simulink model "VCMGCM1962020b_v2"  (R2020b)
settings: Solver=FixedStepDiscrete  StartTime=0.0  StopTime=10.0  FixedStep=0.005  RelTol=1e-3  EnableMultiTasking=on
PreLoadFcn:
  | try, model_open; catch, disp('Error occurred while executing model pre-load callback: model_open.m'); disp('Please assure that the MATLAB working directory is set to the model directory before opening.'); end
InitFcn:
  | try, model_open; catch, end
undefined symbols (not defined in the file): Bridge, GCM, H, raptor_get_param_eval, raptor_get_safe_string, raptor_xcp_function
libraries: Blocks_lib x1165, Raptor_lib x665, simulink x62, VCM_lib x5
(part 2 of 23)

== system VCMGCM1962020b_v2/Fgnd/Diagnostics/Fault Statuses ==
  Data : Inport
  Clear All Faults : Subsystem
  Drive Cycle Logic : Subsystem
  FCC(w/Inpt) : Blocks_lib/FCC(w//Inpt)  SystemSampleTime=-1  VariantActivationTime=update diagram  Latency=0  AutoFrameSizeCalculation=off
  FltStatuses : Blocks_lib/FltStatuses  nam='Fault1'  group=[group ' | Fault1']
  FltStatuses1 : Blocks_lib/FltStatuses  nam='Fault2'  group=[group ' | Fault2']
  FltStatuses2 : Blocks_lib/FltStatuses  nam='Fault3'  group=[group ' | Fault3']
  Header : Blocks_lib/Header  width=Portrait  addtext=''
  Save NV : Subsystem
  Status Marquees : Subsystem
  raptor_adjustment : Raptor_lib/Data Storage/raptor_adjustment  paramName='FaultMarqueeRate'  nameSource=Parameter  initValue=1/samptime  dataType=uint16  storage=Calibration  calDispType=Number  calEnum={'Disabled', 'Enabled'}  calGain=samptime  calOffset=0  calMax=inf  calMin=-inf  calFormat='0.3'  calUnit='sec'  calHelp='Fault marquee update rate'  calAccess=1  calFunction=group  calDispHeaders=off  calColHeaders={'Col1' 'Col2' 'Col3'}  calRowHeaders={'Row1' 'Row2' 'Row3'}
      settings: SourceProductName=Raptor
  raptor_data_def1 : Raptor_lib/Data Storage/raptor_data_def  dataName='ClearFaults'  initValue=0  dataType=boolean  storage=Volatile (RAM)  calVisible=on  calType=Adjustment  calDispType=Enumeration  calEnum={'-', 'Clear'}  calGain=1  calOffset=0  calMin=-inf  calMax=inf  calFormat=''  calUnit='enum'  calHelp='Clear faults'  calAccess=1  calFunction=group  calDispHeaders=off  calColHeaders={'Col1' 'Col2' 'Col3'}  calRowHeaders={'Row1' 'Row2' 'Row3'}
      settings: SourceProductName=Raptor
  raptor_data_def2 : Raptor_lib/Data Storage/raptor_data_def  dataName='SaveNV'  initValue=0  dataType=boolean  storage=Volatile (RAM)  calVisible=on  calType=Adjustment  calDispType=Enumeration  calEnum={'-', 'Save'}  calGain=1  calOffset=0  calMin=-inf  calMax=inf  calFormat=''  calUnit='enum'  calHelp='Save nonvolatile'  calAccess=1  calFunction=group  calDispHeaders=off  calColHeaders={'Col1' 'Col2' 'Col3'}  calRowHeaders={'Row1' 'Row2' 'Row3'}
      settings: SourceProductName=Raptor
  raptor_data_read : Raptor_lib/Data Storage/raptor_data_read  dataName='ClearFaults'  dataShape=Scalar  idxSource=Input  idxRow=1  idxCol=1
      settings: SourceProductName=Raptor
  raptor_data_read1 : Raptor_lib/Data Storage/raptor_data_read  dataName='SaveNV'  dataShape=Scalar  idxSource=Input  idxRow=1  idxCol=1
      settings: SourceProductName=Raptor
  raptor_measurement : Raptor_lib/Data Storage/raptor_measurement  paramName='NVStoreInProgress'  nameSource=Parameter  calDispType=Number  calEnum={'Disabled', 'Enabled'}  calGain=1  calOffset=0  calMax=inf  calMin=-inf  calFormat=''  calUnit='Bool'  calHelp='Nonvolatile store in progress'  calAccess=1  calFunction='Diagnostics | Fault Statuses'  calVisible=on
      settings: SourceProductName=Raptor
  raptor_measurement1 : Raptor_lib/Data Storage/raptor_measurement  paramName='NVSucceeded'  nameSource=Parameter  calDispType=Number  calEnum={'Disabled', 'Enabled'}  calGain=1  calOffset=0  calMax=inf  calMin=-inf  calFormat=''  calUnit='Bool'  calHelp='Nonvolatile store succeeded'  calAccess=1  calFunction='Diagnostics | Fault Statuses'  calVisible=on
      settings: SourceProductName=Raptor
  raptor_sfun_nv_status : Raptor_lib/Data Storage/raptor_sfun_nv_status  showStatus=Store In Progess
      settings: SourceProductName=Raptor
  raptor_sfun_nv_status1 : Raptor_lib/Data Storage/raptor_sfun_nv_status  showStatus=Store Succeeded
      settings: SourceProductName=Raptor
  wires:
  raptor_adjustment/1 -> FCC(w/Inpt)/1
  raptor_data_read/1 -> Clear All Faults/Enable
  raptor_data_read1/1 -> Save NV/Enable
  FCC(w/Inpt)/1 -> Status Marquees/Trigger
  Data/1 -> Drive Cycle Logic/1(Data)
  raptor_sfun_nv_status/1 -> raptor_measurement/1
  raptor_sfun_nv_status1/1 -> raptor_measurement1/1

== system VCMGCM1962020b_v2/Fgnd/Sensors/CAN ==
  Data : Inport
  Battery : Subsystem  mask{bus='CAN1'}
      mask prompts: bus "CAN Bus"
      mask Display: disp(['BMS: Battery\n' bus]);
  Bus Creator : BusCreator  Inputs=5
  CCS Interface : Subsystem  Commented=on  mask{nam='CCS', bus='CAN1'}
      mask prompts: nam "Name"; bus "CAN Bus"
      mask Display: disp(['CCS Interface: IoTecha M2iEV\n' nam '\n' bus]);
  Charger : Subsystem  mask{nam='Chgr', bus='CAN1'}
      mask prompts: nam "Name"; bus "CAN Bus"
      mask Display: disp(['On-Board Charger: Dilong\n' nam '\n' bus]);
  DC/DC Converter : Subsystem  mask{nam='DCDC', bus='CAN1'}
      mask prompts: nam "Name"; bus "CAN Bus"
      mask Display: disp(['DC/DC Converter: Dilong\n' nam '\n' bus]);
  Header : Blocks_lib/Header  width=Portrait  addtext=''
  Inverter : Subsystem  mask{bus='CAN3'}
      mask prompts: bus "CAN Bus"
      mask Display: disp(['Sieatta: Invrtr2\n' bus]);
  Other : Subsystem
  CAN : Outport  VectorParamsAs1DForOutWhenUnconnected=off
  wires:
  Inverter/1(CAN) -> Bus Creator/4
  Other/1(CAN) -> Bus Creator/5
  Charger/1(CAN) -> Bus Creator/2
  Battery/1(CAN) -> Bus Creator/1
  Bus Creator/1 -> CAN/1  "CAN"
  Data/1 -> Battery/1(Data), CCS Interface/1(Data), Charger/1(Data), Other/1(Data), Inverter/1(Data), DC/DC Converter/1(Data)
  DC/DC Converter/1(CAN) -> Bus Creator/3

== system VCMGCM1962020b_v2/Fgnd/Sensors/Sensors ==
  Data : Inport
  Bus Creator : BusCreator  Inputs=3
  Driver Inputs : Subsystem
  Header : Blocks_lib/Header  width=Portrait  addtext=''
  Other : Subsystem
  Voltage : Subsystem
  Sns : Outport  VectorParamsAs1DForOutWhenUnconnected=off
  wires:
  Other/1(Sns) -> Bus Creator/3
  Driver Inputs/1(Sns) -> Bus Creator/2
  Voltage/1(Sns) -> Bus Creator/1
  Bus Creator/1 -> Sns/1  "Sensors"
  Data/1 -> Voltage/1(Data), Other/1(Data), Driver Inputs/1(Data)

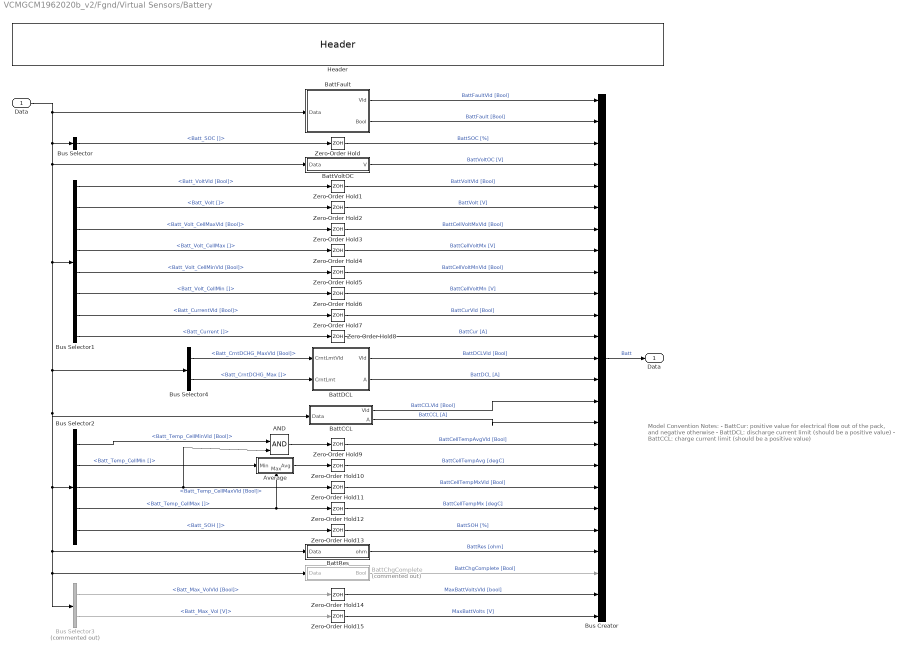
== system VCMGCM1962020b_v2/Fgnd/Virtual Sensors/Battery ==
  note: Model Convention Notes:
      | - BattCur: positive value for electrical flow out of the pack, and negative otherwise
      | - BattDCL: discharge current limit (should be a positive value)
      | - BattCCL: charge current limit (should be a positive value)
  Data : Inport
  AND : Logic  IconShape=distinctive  AllPortsSameDT=off  OutDataTypeStr=boolean
  Average : Subsystem
      settings: PortSchema="{\"entries\":[{\"content\":{\"sides\":[{\"content\":{\"connectorIds\":[\"In1\"]},\"type\":\"ConnectorPlacement.EquallySpacedRectSide\",\"uuid\":\"d9ce9f9a-84a0-4d2c-b22c-bde2c1e2d059\"},{\"content\":{\"connectorIds\":[\"Out1\"],\"side\":\"RIGHT\"},\"type\":\"ConnectorPlacement.EquallySpacedRectSide\",\"uuid\":\"15af732b-6599-4303-92ae-4f716d2d6ef7\"},{\"content\":{\"connectorIds\":[],\"side\":\"TOP\"},\"type\":\"ConnectorPlacement.EquallySpacedRectSide\",\"uuid\":\"c502e606-7455-4b79-ae1a-42fe114835b7\"},{\"content\":{\"connectorIds\":[\"In2\"],\"side\":\"BOTTOM\"},\"type\":\"ConnectorPlacement.EquallySpacedRectSide\",\"uuid\":\"09754e92-d425-4c42-b1f4-651282dd1591\"},{\"content\":{\"connectorIds\":[],\"side\":\"HIDDEN\"},\"type\":\"ConnectorPlacement.EquallySpacedRectSide\",\"uuid\":\"b5cad8d8-bd34-4b5c-af02-955cb15cf870\"}]},\"type\":\"ConnectorPlacement.EquallySpacedConnector\",\"uuid\":\"2eb02162-2dec-4f79-8472-1f908402e422\"}],\"packageUris\":[\"http://schema.mathworks.com/mf0/Connector/R2020b\"],\"version\":\"1.0\"}"
  BattCCL : Subsystem
  BattChgComplete : Subsystem  Commented=on
  BattDCL : Subsystem
  BattFault : Subsystem
  BattRes : Subsystem
  BattVoltOC : Subsystem
  Bus Creator : BusCreator  Inputs=25
  Bus Selector : BusSelector  OutputSignals=Sensors.CAN.Batt.BMS2_VoltageSOC.Batt_SOC.Batt_SOC []
  Bus Selector1 : BusSelector  OutputSignals=Sensors.CAN.Batt.BMS2_VoltageSOC.Batt_Volt.Batt_VoltVld [Bool],Sensors.CAN.Batt.BMS2_VoltageSOC.Batt_Volt.Batt_Volt [],Sensors.CAN.Batt.BMS3_Cell.Batt_Volt_CellMax.Batt_Volt_CellMaxVld [Bool],Sensors.CAN.Batt.BMS3_Cell.Batt_Volt_CellMax.Batt_Volt_CellMax [],Sensors.CAN.Batt.BMS3_Cell.Batt_Volt_CellMin.Batt_Volt_CellMinVld [Bool],Sensors.CAN.Batt.BMS3_Cell.Batt_Volt_CellMin.Batt_Volt_CellMin [],Sensors.CAN.Batt.BMS1_Currents.Batt_Current.Batt_CurrentVld [Bool],Sensors.CAN.Batt.BMS1_Currents.Batt_Current.Batt_Current []
  Bus Selector2 : BusSelector  OutputSignals=Sensors.CAN.Batt.BMS3_Cell.Batt_Temp_CellMin.Batt_Temp_CellMinVld [Bool],Sensors.CAN.Batt.BMS3_Cell.Batt_Temp_CellMin.Batt_Temp_CellMin [],Sensors.CAN.Batt.BMS3_Cell.Batt_Temp_CellMax.Batt_Temp_CellMaxVld [Bool],Sensors.CAN.Batt.BMS3_Cell.Batt_Temp_CellMax.Batt_Temp_CellMax [],Sensors.CAN.Batt.BMS2_VoltageSOC.Batt_SOH.Batt_SOH []
  Bus Selector3 : BusSelector  Commented=on  OutputSignals=Sensors.CAN.Batt.HVES1_Data7.Batt_Max_Vol.Batt_Max_VolVld [Bool],Sensors.CAN.Batt.HVES1_Data7.Batt_Max_Vol.Batt_Max_Vol [V]
  Bus Selector4 : BusSelector  OutputSignals=Sensors.CAN.Batt.BMS1_Currents.Batt_CrntDCHG_Max.Batt_CrntDCHG_MaxVld [Bool],Sensors.CAN.Batt.BMS1_Currents.Batt_CrntDCHG_Max.Batt_CrntDCHG_Max []
  Header : Blocks_lib/Header  width=Portrait  addtext=''
  Zero-Order Hold{,1..15} (16 alike) : ZeroOrderHold  SampleTime=-1
  " Data" : Outport  VectorParamsAs1DForOutWhenUnconnected=off
  wires:
  Zero-Order Hold13/1 -> Bus Creator/21  "BattSOH [%]"
  BattRes/1(ohm) -> Bus Creator/22  "BattRes [ohm]"
  BattChgComplete/1(Bool) -> Bus Creator/23  "BattChgComplete [Bool]"
  Zero-Order Hold12/1 -> Bus Creator/20  "BattCellTempMx [degC]"
  Zero-Order Hold10/1 -> Bus Creator/18  "BattCellTempAvg [degC]"
  BattCCL/2(A) -> Bus Creator/16  "BattCCL [A]"
  BattDCL/2(A) -> Bus Creator/14  "BattDCL [A]"
  Zero-Order Hold8/1 -> Bus Creator/12  "BattCur [A]"
  Zero-Order Hold6/1 -> Bus Creator/10  "BattCellVoltMn [V]"
  Zero-Order Hold4/1 -> Bus Creator/8  "BattCellVoltMx [V]"
  Zero-Order Hold2/1 -> Bus Creator/6  "BattVolt [V]"
  Bus Creator/1 -> " Data"/1  "Batt"
  Zero-Order Hold/1 -> Bus Creator/3  "BattSOC [%]"
  Bus Selector/1 -> Zero-Order Hold/1  "<Batt_SOC []>"
  BattVoltOC/1(V) -> Bus Creator/4  "BattVoltOC [V]"
  Data/1 -> BattVoltOC/1(Data), BattRes/1(Data), Bus Selector3/1, BattChgComplete/1(Data), Bus Selector2/1, BattCCL/1(Data), Bus Selector4/1, Bus Selector1/1, Bus Selector/1, BattFault/1(Data)
  BattFault/1(Vld) -> Bus Creator/1  "BattFaultVld [Bool]"
  Zero-Order Hold1/1 -> Bus Creator/5  "BattVoltVld [Bool]"
  Bus Selector1/7 -> Zero-Order Hold7/1  "<Batt_CurrentVld [Bool]>"
  Bus Selector1/6 -> Zero-Order Hold6/1  "<Batt_Volt_CellMin []>"
  Bus Selector1/5 -> Zero-Order Hold5/1  "<Batt_Volt_CellMinVld [Bool]>"
  Bus Selector1/4 -> Zero-Order Hold4/1  "<Batt_Volt_CellMax []>"
  Bus Selector1/3 -> Zero-Order Hold3/1  "<Batt_Volt_CellMaxVld [Bool]>"
  Bus Selector1/2 -> Zero-Order Hold2/1  "<Batt_Volt []>"
  Bus Selector1/1 -> Zero-Order Hold1/1  "<Batt_VoltVld [Bool]>"
  Zero-Order Hold3/1 -> Bus Creator/7  "BattCellVoltMxVld [Bool]"
  Zero-Order Hold5/1 -> Bus Creator/9  "BattCellVoltMnVld [Bool]"
  Zero-Order Hold7/1 -> Bus Creator/11  "BattCurVld [Bool]"
  BattDCL/1(Vld) -> Bus Creator/13  "BattDCLVld [Bool]"
  BattCCL/1(Vld) -> Bus Creator/15  "BattCCLVld [Bool]"
  Zero-Order Hold9/1 -> Bus Creator/17  "BattCellTempAvgVld [Bool]"
  Zero-Order Hold11/1 -> Bus Creator/19  "BattCellTempMxVld [Bool]"
  BattFault/2(Bool) -> Bus Creator/2  "BattFault [Bool]"
  Bus Selector3/1 -> Zero-Order Hold14/1  "<Batt_Max_VolVld [Bool]>"
  Bus Selector3/2 -> Zero-Order Hold15/1  "<Batt_Max_Vol [V]>"
  Zero-Order Hold15/1 -> Bus Creator/25  "MaxBattVolts [V]"
  Zero-Order Hold14/1 -> Bus Creator/24  "MaxBattVoltsVld [bool]"
  AND/1 -> Zero-Order Hold9/1
  Bus Selector2/1 -> AND/1  "<Batt_Temp_CellMinVld [Bool]>"
  Bus Selector2/2 -> Average/1(Min)  "<Batt_Temp_CellMin []>"
  Bus Selector2/3 -> AND/2, Zero-Order Hold11/1  "<Batt_Temp_CellMaxVld [Bool]>"
  Bus Selector2/4 -> Zero-Order Hold12/1, Average/2(Max)  "<Batt_Temp_CellMax []>"
  Bus Selector2/5 -> Zero-Order Hold13/1  "<Batt_SOH []>"
  Average/1(Avg) -> Zero-Order Hold10/1
  Bus Selector4/1 -> BattDCL/1(CrntLmtVld)  "<Batt_CrntDCHG_MaxVld [Bool]>"
  Bus Selector4/2 -> BattDCL/2(CrntLmt)  "<Batt_CrntDCHG_Max []>"
  Bus Selector1/8 -> Zero-Order Hold8/1  "<Batt_Current []>"

== system VCMGCM1962020b_v2/Fgnd/Virtual Sensors/Charger ==
  Data : Inport
  Bus Creator : BusCreator  Inputs=4
  ChgPlugState : Subsystem
  ChgPortDCVolt : Subsystem
  Header : Blocks_lib/Header  width=Portrait  addtext=''
  Off Board : Subsystem  Commented=on
  On Board : Subsystem
  " Data" : Outport  VectorParamsAs1DForOutWhenUnconnected=off
  wires:
  Bus Creator/1 -> " Data"/1  "Chgr"
  ChgPlugState/1(enum) -> Bus Creator/1  "ChgPlugState [enum]"
  On Board/1(" Data") -> Bus Creator/4  "OnBoard"
  ChgPortDCVolt/1(Vld) -> Bus Creator/2  "ChgPortDCVoltVld [Bool]"
  ChgPortDCVolt/2(V) -> Bus Creator/3  "ChgPortDCVolt [V]"
  Data/1 -> ChgPlugState/1(Data), On Board/1(Data), Off Board/1(Data), ChgPortDCVolt/1(Data)

== system VCMGCM1962020b_v2/Fgnd/Virtual Sensors/DC//DC Converter ==
  Data : Inport
  Bus Creator : BusCreator  Inputs=6
  Bus Selector : BusSelector  OutputSignals=Sensors.CAN.DCDC.DCDC_Status_0_16V.DCDCOutput_Voltage_0_16V.DCDCOutput_Voltage_0_16VVld [Bool],Sensors.CAN.DCDC.DCDC_Status_0_16V.DCDCOutput_Voltage_0_16V.DCDCOutput_Voltage_0_16V [V]
  Bus Selector1 : BusSelector  OutputSignals=Sensors.CAN.DCDC.DCDC_Status_0_16V.DCDC_Inner_temp_0_16V.DCDC_Inner_temp_0_16V [C]
  DCDCFault : Subsystem
  DCDCInptCur : Subsystem
  Header : Blocks_lib/Header  width=Portrait  addtext=''
  Zero-Order Hold : ZeroOrderHold  SampleTime=-1
  Zero-Order Hold1 : ZeroOrderHold  SampleTime=-1
  Zero-Order Hold2 : ZeroOrderHold  SampleTime=-1
  " Data" : Outport  VectorParamsAs1DForOutWhenUnconnected=off
  wires:
  Bus Creator/1 -> " Data"/1  "DCDC"
  Zero-Order Hold2/1 -> Bus Creator/6  "DCDCTemp [degC]"
  Zero-Order Hold1/1 -> Bus Creator/4  "DCDCInptVolt [V]"
  Bus Selector1/1 -> Zero-Order Hold2/1  "<DCDC_Inner_temp_0_16V [C]>"
  Bus Selector/2 -> Zero-Order Hold1/1  "<DCDCOutput_Voltage_0_16V [V]>"
  Zero-Order Hold/1 -> Bus Creator/3  "DCDCInptVoltVld [Bool]"
  Bus Selector/1 -> Zero-Order Hold/1  "<DCDCOutput_Voltage_0_16VVld [Bool]>"
  DCDCFault/1(Vld) -> Bus Creator/1  "DCDCFaultVld [Bool]"
  Data/1 -> DCDCFault/1(Data), Bus Selector/1, Bus Selector1/1, DCDCInptCur/1(Data)
  DCDCFault/2(Bool) -> Bus Creator/2  "DCDCFault [Bool]"
  DCDCInptCur/1(A) -> Bus Creator/5  "DCDCInptCur [A]"

== system VCMGCM1962020b_v2/Fgnd/Virtual Sensors/Drive Inverter ==
  note: TBC
  note: Model Convention Notes:
      | - InvtrCur: positive value for electrical flow into the inverter, and negative otherwise
      | - MtrTrq: may be positive or negative (motoring when torque and speed have same signs; generating when torque and speed have opposite signs)
      | - MtrTrqLimMx: limit on torque in positive speed direction (should be a positive value)
      | - MtrTrqLimMn: limit on torque in negative speed direction (should be a negative value)
  Data : Inport
  Bus Creator : BusCreator  Inputs=16
  Bus Selector : BusSelector  OutputSignals=Sensors.CAN.DrvInvtr.EM3.EM3DCv.EM3_InverterDcV.EM3_InverterDcVVld [Bool],Sensors.CAN.DrvInvtr.EM3.EM3DCv.EM3_InverterDcV.EM3_InverterDcV [V]
  Bus Selector1 : BusSelector  OutputSignals=Sensors.CAN.DrvInvtr.EM2.EM2Invemp.EM2_InverterBridgeMaxTemp.EM2_InverterBridgeMaxTemp [degC],Sensors.CAN.DrvInvtr.EM4.EM4Spd.EM4_SpdAct.EM4_SpdActVld [Bool],Sensors.CAN.DrvInvtr.EM4.EM4Spd.EM4_SpdAct.EM4_SpdAct [rpm],Sensors.CAN.DrvInvtr.EM4.EM4Trq.EM4_TorqAct.EM4_TorqActVld [Bool],Sensors.CAN.DrvInvtr.EM4.EM4Trq.EM4_TorqAct.EM4_TorqAct [Nm],Sensors.CAN.DrvInvtr.EM1.EM1_eBridgeOvrTemp.EM1_eBridgeOvrTempVld [Bool],Sensors.CAN.DrvInvtr.EM1.EM1_eMotorOvrTemp.EM1_eMotorOvrTemp []
  Constant : Constant  Value=double(99999)
  DrvInvtrCur : Subsystem
  DrvInvtrFault : Subsystem
  DrvMtrTmp : Subsystem
  Gain : Gain  Gain=-1
  Header : Blocks_lib/Header  width=Portrait  addtext=''
  Zero-Order Hold{,1..10} (11 alike) : ZeroOrderHold  SampleTime=-1
  " Data" : Outport  VectorParamsAs1DForOutWhenUnconnected=off
  wires:
  Bus Creator/1 -> " Data"/1  "DrvInvtr"
  Zero-Order Hold1/1 -> Bus Creator/4  "DrvInvtrVolt [V]"
  Zero-Order Hold2/1 -> Bus Creator/7  "DrvInvtrTemp [degC]"
  DrvMtrTmp/1(degC) -> Bus Creator/16  "DrvMtrTemp [degC]"
  Zero-Order Hold8/1 -> Bus Creator/13  "DrvMtrTrqLimMn [Nm]"
  Zero-Order Hold4/1 -> Bus Creator/9  "DrvMtrSpd [rpm]"
  Zero-Order Hold7/1 -> Bus Creator/12  "DrvMtrTrqLimMx [Nm]"
  Bus Selector/2 -> Zero-Order Hold1/1  "<EM3_InverterDcV [V]>"
  Constant/1 -> Gain/1, Zero-Order Hold7/1  "<DrvInvtrNegativeTorqueAvailable [Nm]>"
  Zero-Order Hold6/1 -> Bus Creator/11  "DrvMtrTrq [Nm]"
  Zero-Order Hold5/1 -> Bus Creator/10  "DrvMtrTrqVld [Bool]"
  Bus Selector/1 -> Zero-Order Hold/1  "<EM3_InverterDcVVld [Bool]>"
  Zero-Order Hold/1 -> Bus Creator/3  "DrvInvtrVoltVld [Bool]"
  DrvInvtrCur/1(Vld) -> Bus Creator/5  "DrvInvtrCurVld [Bool]"
  DrvInvtrFault/1(Vld) -> Bus Creator/1  "DrvInvtrFaultVld [Bool]"
  Data/1 -> DrvInvtrFault/1(Data), Bus Selector/1, DrvMtrTmp/1(Data), Bus Selector1/1, DrvInvtrCur/1(Data)
  Zero-Order Hold3/1 -> Bus Creator/8  "DrvMtrSpdVld [Bool]"
  DrvInvtrFault/2(Bool) -> Bus Creator/2  "DrvInvtrFault [Bool]"
  DrvInvtrCur/2(A) -> Bus Creator/6  "DrvInvtrCur [A]"
  Gain/1 -> Zero-Order Hold8/1
  Zero-Order Hold9/1 -> Bus Creator/14  "DrvInvtrOvrTemp [Bool]"
  Zero-Order Hold10/1 -> Bus Creator/15  "DrvMtrOvrTemp [Bool]"
  Bus Selector1/1 -> Zero-Order Hold2/1  "<EM2_InverterBridgeMaxTemp [degC]>"
  Bus Selector1/2 -> Zero-Order Hold3/1  "<EM4_SpdActVld [Bool]>"
  Bus Selector1/3 -> Zero-Order Hold4/1  "<EM4_SpdAct [rpm]>"
  Bus Selector1/4 -> Zero-Order Hold5/1  "<EM4_TorqActVld [Bool]>"
  Bus Selector1/5 -> Zero-Order Hold6/1  "<EM4_TorqAct [Nm]>"
  Bus Selector1/6 -> Zero-Order Hold9/1  "<EM1_eBridgeOvrTempVld [Bool]>"
  Bus Selector1/7 -> Zero-Order Hold10/1  "<EM1_eMotorOvrTemp []>"

== system VCMGCM1962020b_v2/Fgnd/Virtual Sensors/Driver Inputs ==
  Data : Inport
  APP : Subsystem
  Brk : Subsystem
  Bus Creator : BusCreator  Inputs=15
  Bus Selector : BusSelector  OutputSignals=Sensors.Sensors.Driver.Rev.Rev [Bool],Sensors.Sensors.Driver.Ntrl.Ntrl [Bool],Sensors.Sensors.Driver.Drv.Drv [Bool],Sensors.Sensors.Driver.CCOn.CCOn [Bool],Sensors.Sensors.Driver.CCCancel.CCCancel [Bool],Sensors.Sensors.Driver.CCSetCst.CCSetCst [Bool],Sensors.Sensors.Driver.CCRsmAcc.CCRsmAcc [Bool]
  Header : Blocks_lib/Header  width=Portrait  addtext=''
  NOR : Logic  Operator=NOR  AllPortsSameDT=off  OutDataTypeStr=boolean
  ParkBrake : Subsystem
  Terminator : Terminator
  VehPwrMode : Subsystem
  Zero-Order Hold{1..8} (8 alike) : ZeroOrderHold  SampleTime=-1
  " Data" : Outport  VectorParamsAs1DForOutWhenUnconnected=off
  wires:
  APP/1(Vld) -> Bus Creator/2  "APPVld [Bool]"
  Bus Selector/6 -> Zero-Order Hold7/1  "<CCSetCst [Bool]>"
  Bus Selector/5 -> Zero-Order Hold6/1  "<CCCancel [Bool]>"
  Bus Selector/4 -> Zero-Order Hold5/1  "<CCOn [Bool]>"
  Bus Selector/3 -> NOR/2, Zero-Order Hold4/1  "<Drv [Bool]>"
  Bus Selector/1 -> Zero-Order Hold2/1, NOR/1  "<Rev [Bool]>"
  Data/1 -> VehPwrMode/1(Data), ParkBrake/1(Data), Bus Selector/1, Brk/1(Data), APP/1(Data)
  Bus Creator/1 -> " Data"/1  "Driver"
  Zero-Order Hold6/1 -> Bus Creator/13  "CCCancel [Bool]"
  Zero-Order Hold5/1 -> Bus Creator/12  "CCOn [Bool]"
  Zero-Order Hold8/1 -> Bus Creator/15  "CCRsmAcc [Bool]"
  Zero-Order Hold7/1 -> Bus Creator/14  "CCSetCst [Bool]"
  Zero-Order Hold4/1 -> Bus Creator/11  "Drv [Bool]"
  Zero-Order Hold3/1 -> Bus Creator/10  "Ntrl [Bool]"
  Zero-Order Hold2/1 -> Bus Creator/9  "Rev [Bool]"
  Zero-Order Hold1/1 -> Bus Creator/8  "Prk [Bool]"
  VehPwrMode/1(enum) -> Bus Creator/1  "VehPwrMode [enum]"
  APP/2(%) -> Bus Creator/3  "APP [%]"
  Brk/2(Brk) -> Bus Creator/5  "BrkSw [Bool]"
  Bus Selector/7 -> Zero-Order Hold8/1  "<CCRsmAcc [Bool]>"
  Brk/1(Vld) -> Bus Creator/4  "BrkVld [Bool]"
  Brk/3(Pos) -> Bus Creator/6  "BrkPos [%]"
  Brk/4(PosVld) -> Bus Creator/7  "BrkPosVld [Bool]"
  NOR/1 -> Zero-Order Hold3/1
  Bus Selector/2 -> Terminator/1  "<Ntrl [Bool]>"
  ParkBrake/1(Prk) -> Zero-Order Hold1/1

== system VCMGCM1962020b_v2/Fgnd/Virtual Sensors/Other ==
  Data : Inport
  Bus Creator : BusCreator  Inputs=7
  Bus Selector : BusSelector  OutputSignals=Sensors.Sensors.Driver.ACSw.ACSw [Bool],Sensors.Sensors.Other.ACPress.ACPress [kPa],Sensors.Sensors.Other.ACEvapTemp.ACEvapTemp [degC],Sensors.Sensors.Other.AmbientAirTemp.AmbientAirTemp [degC],Sensors.Sensors.Driver.HeaterSw.HeaterSw [Bool],Sensors.Sensors.Other.CoolTemp1.CoolTemp1 [degC],Sensors.Sensors.Other.CoolTemp2.CoolTemp2 [degC]
  Header : Blocks_lib/Header  width=Portrait  addtext=''
  Zero-Order Hold{,1..6} (7 alike) : ZeroOrderHold  SampleTime=-1
  " Data" : Outport  VectorParamsAs1DForOutWhenUnconnected=off
  wires:
  Data/1 -> Bus Selector/1
  Bus Creator/1 -> " Data"/1  "Other"
  Zero-Order Hold/1 -> Bus Creator/1  "ACCReq [Bool]"
  Zero-Order Hold1/1 -> Bus Creator/2  "ACPress [kPa]"
  Zero-Order Hold2/1 -> Bus Creator/3  "ACEvapTemp [degC]"
  Zero-Order Hold4/1 -> Bus Creator/5  "HeaterReq [Bool]"
  Zero-Order Hold5/1 -> Bus Creator/6  "CoolTemp1 [degC]"
  Zero-Order Hold6/1 -> Bus Creator/7  "CoolTemp2 [degC]"
  Zero-Order Hold3/1 -> Bus Creator/4  "AmbientAirTemp [degC]"
  Bus Selector/3 -> Zero-Order Hold2/1  "<ACEvapTemp [degC]>"
  Bus Selector/4 -> Zero-Order Hold3/1  "<AmbientAirTemp [degC]>"
  Bus Selector/2 -> Zero-Order Hold1/1  "<ACPress [kPa]>"
  Bus Selector/5 -> Zero-Order Hold4/1  "<HeaterSw [Bool]>"
  Bus Selector/1 -> Zero-Order Hold/1  "<ACSw [Bool]>"
  Bus Selector/6 -> Zero-Order Hold5/1  "<CoolTemp1 [degC]>"
  Bus Selector/7 -> Zero-Order Hold6/1  "<CoolTemp2 [degC]>"

== system VCMGCM1962020b_v2/Fgnd/Virtual Sensors/PDU ==
  Data : Inport
  Bus Creator : BusCreator  Inputs=20
  Bus Selector : BusSelector  Commented=on  OutputSignals=Sensors.CAN.Batt.HVES1_Status1.POS_Contact_State.POS_Contact_StateVld [Bool],Sensors.CAN.Batt.HVES1_Status1.POS_Contact_State.POS_Contact_State []
  Bus Selector1 : BusSelector  OutputSignals=Sensors.Sensors.Other.DCDCCntrClosed.DCDCCntrClosedVld [Bool],Sensors.Sensors.Other.DCDCCntrClosed.DCDCCntrClosed [Bool],Sensors.Sensors.Other.ChrgrCntrClosed.ChrgrCntrClosedVld [Bool],Sensors.Sensors.Other.ChrgrCntrClosed.ChrgrCntrClosed [Bool]
  Constant : Constant
  Ground : Ground
  HVAccCur : Subsystem
  HVBusIso : Subsystem  Commented=on
  HVBusVolt : Subsystem
  Header : Blocks_lib/Header  width=Portrait  addtext=''
  MainCntrClosed : Subsystem
  Relational Operator : RelationalOperator  Operator===  OutDataTypeStr=boolean  RndMeth=Simplest
  Zero-Order Hold{,1..11} (12 alike) : ZeroOrderHold  SampleTime=-1
  " Data" : Outport  VectorParamsAs1DForOutWhenUnconnected=off
  wires:
  Bus Creator/1 -> " Data"/1  "PDU"
  Zero-Order Hold11/1 -> Bus Creator/14  "DrvInvtrCntrClosed [Bool]"
  Zero-Order Hold9/1 -> Bus Creator/12  "HVDschgCntrClosed [Bool]"
  Zero-Order Hold5/1 -> Bus Creator/8  "DCDCCntrClosed [Bool]"
  Zero-Order Hold1/1 -> Bus Creator/2  "MainPosCntrClosed [Bool]"
  Zero-Order Hold3/1 -> Bus Creator/4  "MainNegCntrClosed [Bool]"
  Zero-Order Hold/1 -> Bus Creator/1  "MainPosCntrClosedVld [Bool]"
  Bus Selector/1 -> Zero-Order Hold2/1, Zero-Order Hold/1  "<POS_Contact_StateVld [Bool]>"
  Bus Selector/2 -> Relational Operator/1  "<POS_Contact_State []>"
  Zero-Order Hold2/1 -> Bus Creator/3  "MainNegCntrClosedVld [Bool]"
  Zero-Order Hold4/1 -> Bus Creator/7  "DCDCCntrClosedVld  [Bool]"
  Zero-Order Hold8/1 -> Bus Creator/11  "HVDschgCntrClosedVld [Bool]"
  Zero-Order Hold10/1 -> Bus Creator/13  "DrvInvtrCntrClosedVld [Bool]"
  HVAccCur/1(A) -> Bus Creator/20  "HVAccCur [A]"
  HVBusVolt/1(Vld) -> Bus Creator/18  "HVBusVoltVld [Bool]"
  HVBusIso/1(Vld) -> Bus Creator/15  "HVBusIsoVld [Bool]"
  Data/1 -> MainCntrClosed/1(Data), HVBusVolt/1(Data), HVAccCur/1(Data), HVBusIso/1(Data), Bus Selector1/1, Bus Selector/1
  MainCntrClosed/1(Vld) -> Bus Creator/5  "MainCntrClosedVld [Bool]"
  Bus Selector1/2 -> Zero-Order Hold5/1  "<DCDCCntrClosed [Bool]>"
  Bus Selector1/1 -> Zero-Order Hold4/1  "<DCDCCntrClosedVld [Bool]>"
  MainCntrClosed/2(Bool) -> Bus Creator/6  "MainCntrClosed [Bool]"
  HVBusIso/2("ISOTst ") -> Bus Creator/16  "HVBusIso []"
  HVBusVolt/2(V) -> Bus Creator/19  "HVBusVolt [V]"
  Bus Selector1/4 -> Zero-Order Hold7/1  "<ChrgrCntrClosed [Bool]>"
  Bus Selector1/3 -> Zero-Order Hold6/1  "<ChrgrCntrClosedVld [Bool]>"
  Ground/1 -> Zero-Order Hold11/1, Zero-Order Hold10/1, Zero-Order Hold9/1, Zero-Order Hold8/1
  Zero-Order Hold6/1 -> Bus Creator/9  "ChrgrCntrClosedVld[Bool]"
  Zero-Order Hold7/1 -> Bus Creator/10  "ChrgrCntrClosed [Bool]"
  Constant/1 -> Relational Operator/2
  Relational Operator/1 -> Zero-Order Hold3/1, Zero-Order Hold1/1
  HVBusIso/3(ISOFailed) -> Bus Creator/17  "ISOFailed [Bool]"

== system VCMGCM1962020b_v2/Fgnd/Virtual Sensors/Vehicle ==
  Data : Inport
  Bus Creator : BusCreator  Inputs=6
  Header : Blocks_lib/Header  width=Portrait  addtext=''
  Range : Subsystem
  VehDir : Subsystem
  VehOdmtr : Subsystem
  VehSpd : Subsystem
  " Data" : Outport  VectorParamsAs1DForOutWhenUnconnected=off
  wires:
  Bus Creator/1 -> " Data"/1  "Spd"
  VehSpd/2(kph) -> Bus Creator/2  "VehSpd [kph]"
  VehOdmtr/2(km) -> Range/1(Odom), Bus Creator/4  "VehOdmtr [km]"
  VehDir/1(enum) -> Bus Creator/6  "VehDir [enum]"
  Data/1 -> VehDir/1(Data), Range/2(Data), VehOdmtr/1(Data), VehSpd/1(Data)
  VehSpd/1(Vld) -> Bus Creator/1  "VehSpdVld [Bool]"
  Range/1(Range) -> Bus Creator/5  "VehRangeEst [km]"
  VehOdmtr/1(Trip) -> Bus Creator/3  "TripDist [km]"

== system VCMGCM1962020b_v2/Power Up_Down/Background/Debounce ==
  note: Set / Reset
  In : Inport
  Add : Sum
  Constant : Constant  Value=double(0)
  Detect Change : simulink/Logic and Bit Operations/Detect Change  vinit=0  OutDataTypeStr=boolean
  Logic : CombinatorialLogic  TruthTable=[0;1;0;0;1;1;0;0]
  Logical Operator1 : Logic  AllPortsSameDT=off  OutDataTypeStr=boolean
  Logical Operator2 : Logic  AllPortsSameDT=off  OutDataTypeStr=boolean
  Logical Operator3 : Logic  Operator=NOT  Inputs=1  AllPortsSameDT=off  OutDataTypeStr=boolean
  Multiport Switch1 : MultiPortSwitch  DataPortOrder=Zero-based contiguous  Inputs=2  zeroidx=on
  Mux1 : Mux  Inputs=3
  Relational Operator : RelationalOperator  OutDataTypeStr=boolean  RndMeth=Nearest
  Relational Operator1 : RelationalOperator  OutDataTypeStr=boolean  RndMeth=Nearest
  Unit Delay : UnitDelay  SampleTime=-1  HasFrameUpgradeWarning=on
  Unit Delay2 : UnitDelay  InitialCondition=1  SampleTime=-1  HasFrameUpgradeWarning=on
  raptor_adjustment3 : Raptor_lib/Data Storage/raptor_adjustment  paramName='WakeHiTimeThr'  nameSource=Parameter  initValue=0.2  dataType=double  storage=Calibration  calDispType=Number  calEnum={'Active Low', 'Active High'}  calGain=1  calOffset=0  calMax=inf  calMin=-inf  calFormat='-1'  calUnit='sec'  calHelp='State high time threshold'  calAccess=1  calFunction=group  calDispHeaders=off  calColHeaders={'Col1' 'Col2' 'Col3'}  calRowHeaders={'Row1' 'Row2' 'Row3'}
      settings: SourceProductName=Raptor
  raptor_adjustment4 : Raptor_lib/Data Storage/raptor_adjustment  paramName='WakeLoTimeThr'  nameSource=Parameter  initValue=0.2  dataType=double  storage=Calibration  calDispType=Number  calEnum={'Active Low', 'Active High'}  calGain=1  calOffset=0  calMax=inf  calMin=-inf  calFormat='-1'  calUnit='sec'  calHelp='State low time threshold'  calAccess=1  calFunction=group  calDispHeaders=off  calColHeaders={'Col1' 'Col2' 'Col3'}  calRowHeaders={'Row1' 'Row2' 'Row3'}
      settings: SourceProductName=Raptor
  raptor_delta_time : Raptor_lib/Triggers/raptor_delta_time  unit=seconds
      settings: SourceProductName=Raptor
  Out : Outport  VectorParamsAs1DForOutWhenUnconnected=off
  wires:
  Detect Change/1 -> Multiport Switch1/1
  Logical Operator3/1 -> Logical Operator2/1
  Relational Operator/1 -> Logical Operator1/2
  Logical Operator2/1 -> Mux1/2
  Logical Operator1/1 -> Mux1/1
  Mux1/1 -> Logic/1
  Unit Delay2/1 -> Mux1/3
  In/1 -> Detect Change/1, Logical Operator1/1, Logical Operator3/1
  Multiport Switch1/1 -> Unit Delay/1, Relational Operator/1, Relational Operator1/1
  Add/1 -> Multiport Switch1/2
  Constant/1 -> Multiport Switch1/3
  Relational Operator1/1 -> Logical Operator2/2
  Logic/1 -> Unit Delay2/1, Out/1
  Unit Delay/1 -> Add/2
  raptor_delta_time/1 -> Add/1
  raptor_adjustment4/1 -> Relational Operator1/2
  raptor_adjustment3/1 -> Relational Operator/2

== system VCMGCM1962020b_v2/Power Up_Down/Background/Raise Shutdown Event ==
  Trigger : TriggerPort  TriggerType=falling  VariantControl=(inherit)
  Constant : Constant  Value=boolean(1)
  Function-Call Generator : simulink/Ports & Subsystems/Function-Call Generator  sample_time=-1  numberOfIterations=1  DisallowWideOutput=off
  raptor_data_def : Raptor_lib/Data Storage/raptor_data_def  dataName='FgndTasksStopped'  initValue=0  dataType=boolean  storage=Volatile (RAM)  calVisible=on  calType=Measurement  calDispType=Number  calEnum={'False', 'True'}  calGain=1.0  calOffset=0  calMin=-Inf  calMax=Inf  calFormat='-1'  calUnit='Bool'  calHelp='Foreground tasks stopped'  calAccess=1  calFunction=group  calDispHeaders=off  calColHeaders={'Col1' 'Col2' 'Col3'}  calRowHeaders={'Row1' 'Row2' 'Row3'}
      settings: SourceProductName=Raptor
  raptor_data_write : Raptor_lib/Data Storage/raptor_data_write  dataName='FgndTasksStopped'  dataShape=Scalar  idxSource=Input Port  idxRow=1  idxCol=1
      settings: SourceProductName=Raptor
  raptor_shutdown : Raptor_lib/Triggers/raptor_shutdown  null=0
      settings: SourceProductName=Raptor
  wires:
  Constant/1 -> raptor_data_write/1
  Function-Call Generator/1 -> raptor_shutdown/Trigger

== system VCMGCM1962020b_v2/Power Up_Down/Background/Raise Startup Event ==
  Enable : EnablePort
  Trigger : TriggerPort  VariantControl=(inherit)
  Function-Call Generator : simulink/Ports & Subsystems/Function-Call Generator  sample_time=-1  numberOfIterations=1  DisallowWideOutput=off
  raptor_startup : Raptor_lib/Triggers/raptor_startup  null=0
      settings: SourceProductName=Raptor
  wires:
  Function-Call Generator/1 -> raptor_startup/Trigger

== system VCMGCM1962020b_v2/Power Up_Down/Background/Store EEPROM ==
  Trigger : TriggerPort  TriggerType=falling  VariantControl=(inherit)
  Function-Call Generator : simulink/Ports & Subsystems/Function-Call Generator  sample_time=-1  numberOfIterations=1  DisallowWideOutput=off
  raptor_store_nv : Raptor_lib/Data Storage/raptor_store_nv  null=0
      settings: SourceProductName=Raptor
  wires:
  Function-Call Generator/1 -> raptor_store_nv/Trigger

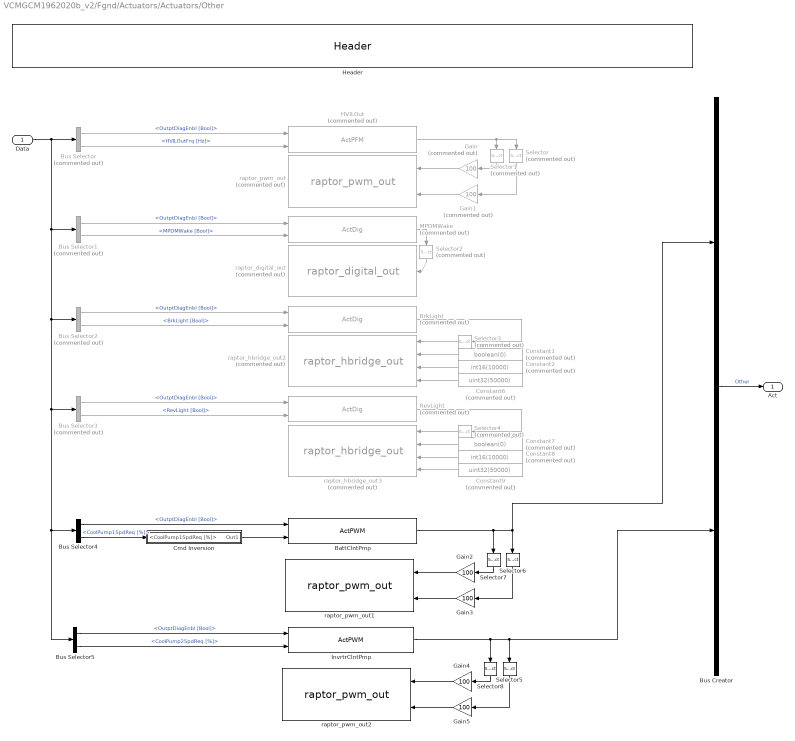
== system VCMGCM1962020b_v2/Fgnd/Actuators/Actuators/Other ==
  Data : Inport
  BattClntPmp : Blocks_lib/ActPWM  text_resource='OUTPUT11'  nam='BattClntPmp'  group='Group'  samptime=samptime
  BrkLight : Blocks_lib/ActDig  Commented=on  text_resource='OUTPUT52_53'  nam='BrkLight'  group='Actuators | Other'  samptime=samptime
  Bus Creator : BusCreator  Inputs=2
  Bus Selector : BusSelector  Commented=on  OutputSignals=Control.Mode.StartStop.OutptDiagEnbl [Bool],Control.Other.Other.HVILOutFrq [Hz]
  Bus Selector1 : BusSelector  Commented=on  OutputSignals=Control.Mode.StartStop.OutptDiagEnbl [Bool],Control.Other.Other.MPDMWake [Bool]
  Bus Selector2 : BusSelector  Commented=on  OutputSignals=Control.Mode.StartStop.OutptDiagEnbl [Bool],Control.Other.Other.Lamp.BrkLight [Bool]
  Bus Selector3 : BusSelector  Commented=on  OutputSignals=Control.Mode.StartStop.OutptDiagEnbl [Bool],Control.Other.Other.Lamp.RevLight [Bool]
  Bus Selector4 : BusSelector  OutputSignals=Control.Mode.StartStop.OutptDiagEnbl [Bool],Control.Other.CoolPump.CoolPump1SpdReq [%]
  Bus Selector5 : BusSelector  OutputSignals=Control.Mode.StartStop.OutptDiagEnbl [Bool],Control.Other.CoolPump.CoolPump2SpdReq [%]
  Cmd Inversion : Subsystem
  Constant1 : Constant  Commented=on  Value=boolean(0)
  Constant2 : Constant  Commented=on  Value=int16(10000)
  Constant6 : Constant  Commented=on  Value=uint32(50000)
  Constant7 : Constant  Commented=on  Value=boolean(0)
  Constant8 : Constant  Commented=on  Value=int16(10000)
  Constant9 : Constant  Commented=on  Value=uint32(50000)
  Gain : Gain  Commented=on  Gain=100  OutDataTypeStr=uint16
  Gain1 : Gain  Commented=on  Gain=100  OutDataTypeStr=uint32
  Gain2 : Gain  Gain=100  OutDataTypeStr=uint16
  Gain3 : Gain  Gain=100  OutDataTypeStr=uint32
  Gain4 : Gain  Gain=100  OutDataTypeStr=uint16
  Gain5 : Gain  Gain=100  OutDataTypeStr=uint32
  HVILOut : Blocks_lib/ActPFM  Commented=on  text_resource='OUTPUT1'  nam='HVILOut'  group='Actuators | Other'  samptime=samptime
  Header : Blocks_lib/Header  width=Portrait  addtext=''
  InvrtrClntPmp : Blocks_lib/ActPWM  text_resource='OUTPUT12'  nam='InvrtrClntPmp'  group='Group'  samptime=samptime
  MPDMWake : Blocks_lib/ActDig  Commented=on  text_resource='OUTPUT30'  nam='MPDMWake'  group='Actuators | Other'  samptime=samptime
  RevLight : Blocks_lib/ActDig  Commented=on  text_resource='OUTPUT54_55'  nam='RevLight'  group='Actuators | Other'  samptime=samptime
  Selector : Selector  Commented=on  InputPortWidth=3  IndexOptions=Index vector (dialog)  Indices=[2]  OutputSizes=1
  Selector1 : Selector  Commented=on  InputPortWidth=3  IndexOptions=Index vector (dialog)  Indices=[3]  OutputSizes=1
  Selector2 : Selector  Commented=on  InputPortWidth=2  IndexOptions=Index vector (dialog)  Indices=[2]  OutputSizes=1
  Selector3 : Selector  Commented=on  InputPortWidth=2  IndexOptions=Index vector (dialog)  Indices=[2]  OutputSizes=1
  Selector4 : Selector  Commented=on  InputPortWidth=2  IndexOptions=Index vector (dialog)  Indices=[2]  OutputSizes=1
  Selector5 : Selector  InputPortWidth=3  IndexOptions=Index vector (dialog)  Indices=[3]  OutputSizes=1
  Selector6 : Selector  InputPortWidth=3  IndexOptions=Index vector (dialog)  Indices=[3]  OutputSizes=1
  Selector7 : Selector  InputPortWidth=3  IndexOptions=Index vector (dialog)  Indices=[2]  OutputSizes=1
  Selector8 : Selector  InputPortWidth=3  IndexOptions=Index vector (dialog)  Indices=[2]  OutputSizes=1
  raptor_digital_out : Raptor_lib/Input & Output/raptor_digital_out  Commented=on  resourceValues=OUTPUT1|OUTPUT2|OUTPUT3|OUTPUT4|OUTPUT5|OUTPUT6|OUTPUT7|OUTPUT8|OUTPUT9|OUTPUT10|OUTPUT11|OUTPUT12|OUTPUT21|OUTPUT22|OUTPUT23|OUTPUT24|OUTPUT25|OUTPUT26|OUTPUT27|OUTPUT28|OUTPUT29|OUTPUT30|OUTPUT31|OUTPUT32|OUTPUT33|OUTPUT34|OUTPUT35|OUTPUT36|OUTPUT37|OUTPUT38|OUTPUT39|OUTPUT40|OUTPUT41|OUTPUT42|OUTPUT43|OUTPUT44|OUTPUT45|OUTPUT46|OUTPUT47|OUTPUT48|OUTPUT49|POWER_HOLD|(None)  resource=OUTPUT30  driverTypeValues=Low Side  driverType=Low Side
      settings: SourceProductName=Raptor
  raptor_hbridge_out2 : Raptor_lib/Input & Output/raptor_hbridge_out  Commented=on  resourceValues=(None)|OUTPUT50_51|OUTPUT52_53|OUTPUT54_55  resource=OUTPUT52_53  outError=0  driverTypeValues=[]  driverType=H-Bridge
      settings: SourceProductName=Raptor
  raptor_hbridge_out3 : Raptor_lib/Input & Output/raptor_hbridge_out  Commented=on  resourceValues=(None)|OUTPUT50_51|OUTPUT52_53|OUTPUT54_55  resource=OUTPUT54_55  outError=0  driverTypeValues=[]  driverType=H-Bridge
      settings: SourceProductName=Raptor
  raptor_pwm_out : Raptor_lib/Input & Output/raptor_pwm_out  Commented=on  showEnable=0  resourceValues=OUTPUT1|OUTPUT2|OUTPUT3|OUTPUT4|OUTPUT5|OUTPUT6|OUTPUT7|OUTPUT8|OUTPUT9|OUTPUT10|OUTPUT11|OUTPUT12|(None)  resource=OUTPUT1  driverTypeValues=Low Side  driverType=Low Side
      settings: SourceProductName=Raptor
  raptor_pwm_out1 : Raptor_lib/Input & Output/raptor_pwm_out  showEnable=0  resourceValues=OUTPUT1|OUTPUT2|OUTPUT3|OUTPUT4|OUTPUT5|OUTPUT6|OUTPUT7|OUTPUT8|OUTPUT9|OUTPUT10|OUTPUT11|OUTPUT12|(None)  resource=OUTPUT8  driverTypeValues=Low Side  driverType=Low Side
      settings: SourceProductName=Raptor
  raptor_pwm_out2 : Raptor_lib/Input & Output/raptor_pwm_out  showEnable=0  resourceValues=OUTPUT1|OUTPUT2|OUTPUT3|OUTPUT4|OUTPUT5|OUTPUT6|OUTPUT7|OUTPUT8|OUTPUT9|OUTPUT10|OUTPUT11|OUTPUT12|(None)  resource=OUTPUT12  driverTypeValues=Low Side  driverType=Low Side
      settings: SourceProductName=Raptor
  Act : Outport  VectorParamsAs1DForOutWhenUnconnected=off
  wires:
  Bus Selector3/1 -> RevLight/1  "<OutptDiagEnbl [Bool]>"
  Constant7/1 -> raptor_hbridge_out3/2
  Selector4/1 -> raptor_hbridge_out3/1
  Gain/1 -> raptor_pwm_out/1
  Selector3/1 -> raptor_hbridge_out2/1
  Selector1/1 -> Gain/1
  Constant9/1 -> raptor_hbridge_out3/4
  Selector/1 -> Gain1/1
  Gain1/1 -> raptor_pwm_out/2
  Bus Selector2/2 -> BrkLight/2  "<BrkLight [Bool]>"
  Bus Selector2/1 -> BrkLight/1  "<OutptDiagEnbl [Bool]>"
  Bus Selector/2 -> HVILOut/2  "<HVILOutFrq [Hz]>"
  Constant2/1 -> raptor_hbridge_out2/3
  Constant6/1 -> raptor_hbridge_out2/4
  Constant8/1 -> raptor_hbridge_out3/3
  BrkLight/1 -> Selector3/1
  Bus Selector/1 -> HVILOut/1  "<OutptDiagEnbl [Bool]>"
  Constant1/1 -> raptor_hbridge_out2/2
  HVILOut/1 -> Selector1/1, Selector/1
  Bus Selector3/2 -> RevLight/2  "<RevLight [Bool]>"
  RevLight/1 -> Selector4/1
  Bus Selector1/1 -> MPDMWake/1  "<OutptDiagEnbl [Bool]>"
  MPDMWake/1 -> Selector2/1
  Bus Selector1/2 -> MPDMWake/2  "<MPDMWake [Bool]>"
  Selector2/1 -> raptor_digital_out/1
  Bus Creator/1 -> Act/1  "Other"
  BattClntPmp/1 -> Bus Creator/1, Selector6/1, Selector7/1
  Bus Selector4/1 -> BattClntPmp/1  "<OutptDiagEnbl [Bool]>"
  Selector6/1 -> Gain3/1
  Gain3/1 -> raptor_pwm_out1/2
  Selector7/1 -> Gain2/1
  Gain2/1 -> raptor_pwm_out1/1
  Gain4/1 -> raptor_pwm_out2/1
  Selector8/1 -> Gain4/1
  Bus Selector5/2 -> InvrtrClntPmp/2  "<CoolPump2SpdReq [%]>"
  InvrtrClntPmp/1 -> Bus Creator/2, Selector5/1, Selector8/1
  Bus Selector5/1 -> InvrtrClntPmp/1  "<OutptDiagEnbl [Bool]>"
  Data/1 -> Bus Selector/1, Bus Selector1/1, Bus Selector5/1, Bus Selector4/1, Bus Selector3/1, Bus Selector2/1
  Gain5/1 -> raptor_pwm_out2/2
  Selector5/1 -> Gain5/1
  Bus Selector4/2 -> Cmd Inversion/1(<CoolPump1SpdReq [%]>)  "<CoolPump1SpdReq [%]>"
  Cmd Inversion/1(Out1) -> BattClntPmp/2

== system VCMGCM1962020b_v2/Fgnd/Actuators/Actuators/PDU ==
  Data : Inport
  Bus Creator : BusCreator  Inputs=5
  Bus Selector : BusSelector  OutputSignals=Control.Mode.StartStop.OutptDiagEnbl [Bool],Control.PDU.PDUCntrs.DCDCCntrCmd [Bool]
  Bus Selector4 : BusSelector  OutputSignals=Control.Mode.StartStop.OutptDiagEnbl [Bool],Control.Mode.StartStop.ChgCntr [Bool]
  Bus Selector5 : BusSelector  Commented=on  OutputSignals=Control.Mode.StartStop.OutptDiagEnbl [Bool],Control.PDU.HVDschgCntr [Bool]
  Bus Selector6 : BusSelector  OutputSignals=Control.Mode.StartStop.OutptDiagEnbl [Bool],Control.PDU.PDUCntrs.DrvInvtrCntrCmd [Bool]
  DCDC_Cntr : Blocks_lib/ActDig  text_resource='OUTPUT22'  nam='DCDC_Cntr'  group='Actuators | PDU'  samptime=samptime
  DrvInvtrCntr : Blocks_lib/ActDig  text_resource='OUTPUT26'  nam='DrvInvtrCntr'  group='Actuators | PDU'  samptime=samptime
  HVDschgCntr : Blocks_lib/ActDig  Commented=on  text_resource='OUTPUT10'  nam='HVDschgCntr'  group='Actuators | PDU'  samptime=samptime
  Header : Blocks_lib/Header  width=Portrait  addtext=''
  OBCCntr : Blocks_lib/ActDig  text_resource='OUTPUT25'  nam='OBCCntr'  group='Actuators | PDU'  samptime=samptime
  PTCHtrCntr : Blocks_lib/ActDig  text_resource='OUTPUT23'  nam='PTCHtrCntr'  group='Actuators | PDU'  samptime=samptime
  PayloadCntr : Blocks_lib/ActDig  text_resource='OUTPUT24'  nam='PayloadCntr'  group='Actuators | PDU'  samptime=samptime
  Selector{,1..2,4,6} (5 alike) : Selector  InputPortWidth=2  IndexOptions=Index vector (dialog)  Indices=[2]  OutputSizes=1
  Selector5 : Selector  Commented=on  InputPortWidth=2  IndexOptions=Index vector (dialog)  Indices=[2]  OutputSizes=1
  raptor_digital_out : Raptor_lib/Input & Output/raptor_digital_out  resourceValues=OUTPUT1|OUTPUT2|OUTPUT3|OUTPUT4|OUTPUT5|OUTPUT6|OUTPUT7|OUTPUT8|OUTPUT9|OUTPUT10|OUTPUT11|OUTPUT12|OUTPUT21|OUTPUT22|OUTPUT23|OUTPUT24|OUTPUT25|OUTPUT26|OUTPUT27|OUTPUT28|OUTPUT29|OUTPUT30|OUTPUT31|OUTPUT32|OUTPUT33|OUTPUT34|OUTPUT35|OUTPUT36|OUTPUT37|OUTPUT38|OUTPUT39|OUTPUT40|OUTPUT41|OUTPUT42|OUTPUT43|OUTPUT44|OUTPUT45|OUTPUT46|OUTPUT47|OUTPUT48|OUTPUT49|POWER_HOLD|(None)  resource=OUTPUT22  driverTypeValues=Low Side  driverType=Low Side
      settings: SourceProductName=Raptor
  raptor_digital_out1 : Raptor_lib/Input & Output/raptor_digital_out  resourceValues=OUTPUT1|OUTPUT2|OUTPUT3|OUTPUT4|OUTPUT5|OUTPUT6|OUTPUT7|OUTPUT8|OUTPUT9|OUTPUT10|OUTPUT11|OUTPUT12|OUTPUT21|OUTPUT22|OUTPUT23|OUTPUT24|OUTPUT25|OUTPUT26|OUTPUT27|OUTPUT28|OUTPUT29|OUTPUT30|OUTPUT31|OUTPUT32|OUTPUT33|OUTPUT34|OUTPUT35|OUTPUT36|OUTPUT37|OUTPUT38|OUTPUT39|OUTPUT40|OUTPUT41|OUTPUT42|OUTPUT43|OUTPUT44|OUTPUT45|OUTPUT46|OUTPUT47|OUTPUT48|OUTPUT49|POWER_HOLD|(None)  resource=OUTPUT23  driverTypeValues=Low Side  driverType=Low Side
      settings: SourceProductName=Raptor
  raptor_digital_out2 : Raptor_lib/Input & Output/raptor_digital_out  resourceValues=OUTPUT1|OUTPUT2|OUTPUT3|OUTPUT4|OUTPUT5|OUTPUT6|OUTPUT7|OUTPUT8|OUTPUT9|OUTPUT10|OUTPUT11|OUTPUT12|OUTPUT21|OUTPUT22|OUTPUT23|OUTPUT24|OUTPUT25|OUTPUT26|OUTPUT27|OUTPUT28|OUTPUT29|OUTPUT30|OUTPUT31|OUTPUT32|OUTPUT33|OUTPUT34|OUTPUT35|OUTPUT36|OUTPUT37|OUTPUT38|OUTPUT39|OUTPUT40|OUTPUT41|OUTPUT42|OUTPUT43|OUTPUT44|OUTPUT45|OUTPUT46|OUTPUT47|OUTPUT48|OUTPUT49|POWER_HOLD|(None)  resource=OUTPUT24  driverTypeValues=Low Side  driverType=Low Side
      settings: SourceProductName=Raptor
  raptor_digital_out4 : Raptor_lib/Input & Output/raptor_digital_out  Commented=on  resourceValues=OUTPUT1|OUTPUT2|OUTPUT3|OUTPUT4|OUTPUT5|OUTPUT6|OUTPUT7|OUTPUT8|OUTPUT9|OUTPUT10|OUTPUT11|OUTPUT12|OUTPUT21|OUTPUT22|OUTPUT23|OUTPUT24|OUTPUT25|OUTPUT26|OUTPUT27|OUTPUT28|OUTPUT29|OUTPUT30|OUTPUT31|OUTPUT32|OUTPUT33|OUTPUT34|OUTPUT35|OUTPUT36|OUTPUT37|OUTPUT38|OUTPUT39|OUTPUT40|OUTPUT41|OUTPUT42|OUTPUT43|OUTPUT44|OUTPUT45|OUTPUT46|OUTPUT47|OUTPUT48|OUTPUT49|POWER_HOLD|(None)  resource=OUTPUT10  driverTypeValues=Low Side  driverType=Low Side
      settings: SourceProductName=Raptor
  raptor_digital_out5 : Raptor_lib/Input & Output/raptor_digital_out  resourceValues=OUTPUT1|OUTPUT2|OUTPUT3|OUTPUT4|OUTPUT5|OUTPUT6|OUTPUT7|OUTPUT8|OUTPUT9|OUTPUT10|OUTPUT11|OUTPUT12|OUTPUT21|OUTPUT22|OUTPUT23|OUTPUT24|OUTPUT25|OUTPUT26|OUTPUT27|OUTPUT28|OUTPUT29|OUTPUT30|OUTPUT31|OUTPUT32|OUTPUT33|OUTPUT34|OUTPUT35|OUTPUT36|OUTPUT37|OUTPUT38|OUTPUT39|OUTPUT40|OUTPUT41|OUTPUT42|OUTPUT43|OUTPUT44|OUTPUT45|OUTPUT46|OUTPUT47|OUTPUT48|OUTPUT49|POWER_HOLD|(None)  resource=OUTPUT26  driverTypeValues=Low Side  driverType=Low Side
      settings: SourceProductName=Raptor
  raptor_digital_out6 : Raptor_lib/Input & Output/raptor_digital_out  resourceValues=OUTPUT1|OUTPUT2|OUTPUT3|OUTPUT4|OUTPUT5|OUTPUT6|OUTPUT7|OUTPUT8|OUTPUT9|OUTPUT10|OUTPUT11|OUTPUT12|OUTPUT21|OUTPUT22|OUTPUT23|OUTPUT24|OUTPUT25|OUTPUT26|OUTPUT27|OUTPUT28|OUTPUT29|OUTPUT30|OUTPUT31|OUTPUT32|OUTPUT33|OUTPUT34|OUTPUT35|OUTPUT36|OUTPUT37|OUTPUT38|OUTPUT39|OUTPUT40|OUTPUT41|OUTPUT42|OUTPUT43|OUTPUT44|OUTPUT45|OUTPUT46|OUTPUT47|OUTPUT48|OUTPUT49|POWER_HOLD|(None)  resource=OUTPUT25  driverTypeValues=Low Side  driverType=Low Side
      settings: SourceProductName=Raptor
  Act : Outport  VectorParamsAs1DForOutWhenUnconnected=off
  wires:
  PayloadCntr/1 -> Bus Creator/3, Selector2/1
  DCDC_Cntr/1 -> Bus Creator/1, Selector/1
  PTCHtrCntr/1 -> Bus Creator/2, Selector1/1
  Bus Creator/1 -> Act/1  "PDU"
  Bus Selector/2 -> PayloadCntr/2, PTCHtrCntr/2, DCDC_Cntr/2  "<DCDCCntrCmd [Bool]>"
  HVDschgCntr/1 -> Selector5/1
  DrvInvtrCntr/1 -> Bus Creator/5, Selector6/1
  OBCCntr/1 -> Bus Creator/4, Selector4/1
  Bus Selector/1 -> PayloadCntr/1, PTCHtrCntr/1, DCDC_Cntr/1  "<OutptDiagEnbl [Bool]>"
  Data/1 -> Bus Selector/1, Bus Selector5/1, Bus Selector6/1, Bus Selector4/1
  Bus Selector4/1 -> OBCCntr/1  "<OutptDiagEnbl [Bool]>"
  Bus Selector4/2 -> OBCCntr/2  "<ChgCntr [Bool]>"
  Bus Selector5/1 -> HVDschgCntr/1  "<OutptDiagEnbl [Bool]>"
  Bus Selector5/2 -> HVDschgCntr/2  "<HVDschgCntr [Bool]>"
  Bus Selector6/1 -> DrvInvtrCntr/1  "<OutptDiagEnbl [Bool]>"
  Bus Selector6/2 -> DrvInvtrCntr/2  "<DrvInvtrCntrCmd [Bool]>"
  Selector/1 -> raptor_digital_out/1
  Selector1/1 -> raptor_digital_out1/1
  Selector2/1 -> raptor_digital_out2/1
  Selector4/1 -> raptor_digital_out6/1
  Selector5/1 -> raptor_digital_out4/1
  Selector6/1 -> raptor_digital_out5/1

== system VCMGCM1962020b_v2/Fgnd/Actuators/CAN/Battery ==
  Data : Inport
  ChgrBatt_State_Transition_Cmd : Subsystem
      mask help:
      | Example of how to set up a CAN message transmit.
      | 1. Copy this block into the main model.
      | 2. Disable/break library link.
      | 3. Underneath, set up CAN Tx Message block.
      | 4. For each field, connect a CANTxField block from the CAN block to the bus creator; adjust parameters as necessary.
      mask init:
      | [msgnam, msgbus] = CANBlockInit('Tx');
      mask Display: disp(['CAN Tx: Message\n' msgnam '\n' msgbus]);
  Ground : Ground
  Header : Blocks_lib/Header  width=Portrait  addtext=''
  MsgName : Subsystem  Commented=on
      mask help:
      | Example of how to set up a CAN message transmit.
      | 1. Copy this block into the main model.
      | 2. Disable/break library link.
      | 3. Underneath, set up CAN Tx Message block.
      | 4. For each field, connect a CANTxField block from the CAN block to the bus creator; adjust parameters as necessary.
      mask init:
      | [msgnam, msgbus] = CANBlockInit('Tx');
      mask Display: disp(['CAN Tx: Message\n' msgnam '\n' msgbus]);
  Act : Outport  VectorParamsAs1DForOutWhenUnconnected=off
  wires:
  Data/1 -> ChgrBatt_State_Transition_Cmd/1(Data), MsgName/1(Data)
  Ground/1 -> Act/1  "Batt"

== system VCMGCM1962020b_v2/Fgnd/Actuators/CAN/Body Control ==
  Data : Inport
  BCMBCH1 : Subsystem
      mask help:
      | Example of how to set up a CAN message transmit.
      | 1. Copy this block into the main model.
      | 2. Disable/break library link.
      | 3. Underneath, set up CAN Tx Message block.
      | 4. For each field, connect a CANTxField block from the CAN block to the bus creator; adjust parameters as necessary.
      mask init:
      | [msgnam, msgbus] = CANBlockInit('Tx');
      mask Display: disp(['CAN Tx: Message\n' msgnam '\n' msgbus]);
  BCMCCVS1_VCU : Subsystem
      mask help:
      | Example of how to set up a CAN message transmit.
      | 1. Copy this block into the main model.
      | 2. Disable/break library link.
      | 3. Underneath, set up CAN Tx Message block.
      | 4. For each field, connect a CANTxField block from the CAN block to the bus creator; adjust parameters as necessary.
      mask init:
      | [msgnam, msgbus] = CANBlockInit('Tx');
      mask Display: disp(['CAN Tx: Message\n' msgnam '\n' msgbus]);
  BCMCM3 : Subsystem
      mask help:
      | Example of how to set up a CAN message transmit.
      | 1. Copy this block into the main model.
      | 2. Disable/break library link.
      | 3. Underneath, set up CAN Tx Message block.
      | 4. For each field, connect a CANTxField block from the CAN block to the bus creator; adjust parameters as necessary.
      mask init:
      | [msgnam, msgbus] = CANBlockInit('Tx');
      mask Display: disp(['CAN Tx: Message\n' msgnam '\n' msgbus]);
  BCMETC2 : Subsystem
      mask help:
      | Example of how to set up a CAN message transmit.
      | 1. Copy this block into the main model.
      | 2. Disable/break library link.
      | 3. Underneath, set up CAN Tx Message block.
      | 4. For each field, connect a CANTxField block from the CAN block to the bus creator; adjust parameters as necessary.
      mask init:
      | [msgnam, msgbus] = CANBlockInit('Tx');
      mask Display: disp(['CAN Tx: Message\n' msgnam '\n' msgbus]);
  BCMICMSTS : Subsystem
      mask help:
      | Example of how to set up a CAN message transmit.
      | 1. Copy this block into the main model.
      | 2. Disable/break library link.
      | 3. Underneath, set up CAN Tx Message block.
      | 4. For each field, connect a CANTxField block from the CAN block to the bus creator; adjust parameters as necessary.
      mask init:
      | [msgnam, msgbus] = CANBlockInit('Tx');
      mask Display: disp(['CAN Tx: Message\n' msgnam '\n' msgbus]);
  BCMVEP2 : Subsystem
      mask help:
      | Example of how to set up a CAN message transmit.
      | 1. Copy this block into the main model.
      | 2. Disable/break library link.
      | 3. Underneath, set up CAN Tx Message block.
      | 4. For each field, connect a CANTxField block from the CAN block to the bus creator; adjust parameters as necessary.
      mask init:
      | [msgnam, msgbus] = CANBlockInit('Tx');
      mask Display: disp(['CAN Tx: Message\n' msgnam '\n' msgbus]);
  Ground : Ground
  Header : Blocks_lib/Header  width=Portrait  addtext=''
  MsgName : Subsystem  Commented=on
      mask help:
      | Example of how to set up a CAN message transmit.
      | 1. Copy this block into the main model.
      | 2. Disable/break library link.
      | 3. Underneath, set up CAN Tx Message block.
      | 4. For each field, connect a CANTxField block from the CAN block to the bus creator; adjust parameters as necessary.
      mask init:
      | [msgnam, msgbus] = CANBlockInit('Tx');
      mask Display: disp(['CAN Tx: Message\n' msgnam '\n' msgbus]);
  Act : Outport  VectorParamsAs1DForOutWhenUnconnected=off
  wires:
  Data/1 -> MsgName/1(Data), BCMCCVS1_VCU/1(Data), BCMVEP2/1(Data), BCMCM3/1(Data), BCMBCH1/1(Data), BCMICMSTS/1(Data), BCMETC2/1(Data)
  Ground/1 -> Act/1  "BCM"
